simulink model "Final_System_Model_V10"  (R2018a)
settings: Solver=VariableStepAuto  StartTime=0  StopTime=250  FixedStep=0.5  RelTol=1e-3
PreLoadFcn:
  | Ts_Power=1e-6;
  | Ts_Control=100e-6;
undefined symbols (not defined in the file): DiscIntNeverNeededParam, sigbuilder_block
libraries: simulink x24, fl_lib x16, powerlib x15, nesl_utility x8, powerlib_meascontrol x5, re_lib x1
(part 1 of 8)
Description:
  | Copyright 2008-2017 The MathWorks, Inc.
settings Model: SimulationMode=accelerator  PacingRate=0.001000  Creator=MathWorks  LastModifiedBy=Mina
settings SolverCC: ZeroCrossControl=EnableAll  ZeroCrossAlgorithm=Adaptive  AlgebraicLoopSolver=LineSearch
settings DataIOCC: LimitDataPoints=on  SaveFormat=Array  SignalLoggingSaveFormat=ModelDataLogs  SignalLogging=off  DSMLogging=off
settings OptimizationCC: ExpressionDepthLimit=2147483647  LifeSpan=inf
settings DebuggingCC: SolverPrmCheckMsg=warning  FcnCallInpInsideContextMsg=warning  StateNameClashWarn=warning  SFUnexpectedBacktrackingDiag=warning  SFNoUnconditionalDefaultTransitionDiag=warning  SFExecutionAtInitializationDiag=none
settings HardwareCC: ProdBitPerPointer=32  ProdBitPerSizeT=32  ProdBitPerPtrDiffT=32  ProdLargestAtomicFloat=None  ProdIntDivRoundTo=Undefined  ProdEndianess=Unspecified  ProdWordSize=32  ProdHWDeviceType=32-bit Generic
settings ModelReferenceCC: PropagateSignalLabelsOutOfModel=off
settings CodeAppCC: StateflowObjectComments=on
settings GRTTargetCC: TargetLangStandard=C89/C90 (ANSI)  GeneratePreprocessorConditionals=Disable all  CombineOutputUpdateFcns=off  GRTInterface=on
settings ConfigComp: CovMetricSettings=dw  CovHtmlReporting=on  CovSaveCumulativeToWorkspaceVar=on  CovSaveSingleToWorkspaceVar=on  CovExternalEMLEnable=off  CovSFcnEnable=off
settings SimscapeCC: SimscapeNormalizeSystem=off

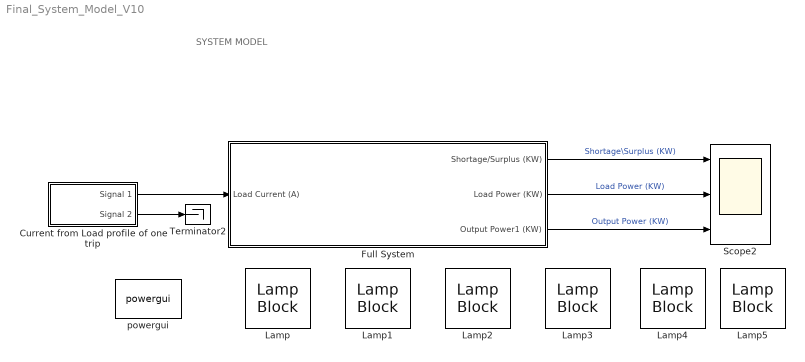
== system Final_System_Model_V10 ==
  note: SYSTEM MODEL
  Current from Load profile of one trip : Subsystem  Tag=STV Subsys  LoadFcn=sigbuilder_block('load');  StartFcn=sigbuilder_block('start');  StopFcn=sigbuilder_block('stop');  ClipboardFcn=sigbuilder_block('clipboard');  mask(Sigbuilder block){tuvar=[0:10]}
      mask help: Simulink:masks:SigbuilderBlock_MD
      mask init:
      | if ~strcmp(get_param(bdroot(gcbh),'SimulationStatus'),'stopped') tuvar = sigbuilder_block('maskInit'); end
      settings: CopyFcn=sigbuilder_block('copy');  DeleteFcn=sigbuilder_block('delete');  ModelCloseFcn=sigbuilder_block('modelClose');  PreSaveFcn=sigbuilder_block('preSave');  PauseFcn=sigbuilder_block('pause');  ContinueFcn=sigbuilder_block('continue');  NameChangeFcn=sigbuilder_block('namechange');  OpenFcn=sigbuilder_block('open',[403.5 117 550.5 359.25 ]);  CloseFcn=sigbuilder_block('close');
      mask Display: plot(0, 0, 100, 100,[2, 2, 32, 32, 2], [68, 8, 8, 68, 68],[32, 2], [38, 38], [32, 19, 2],[53, 60, 44], [32, 17, 17, 2],[16, 16, 31, 31]);txt = getActiveGroup(gcbh);text(2, 100, txt,'verticalAlignment', 'top');
  Full System : Subsystem
  Lamp : LampBlock  WebBlockId=4884
  Lamp1 : LampBlock  WebBlockId=4889
  Lamp2 : LampBlock  WebBlockId=4890
  Lamp3 : LampBlock  WebBlockId=4891
  Lamp4 : LampBlock  WebBlockId=4892
  Lamp5 : LampBlock  WebBlockId=4893
  Scope2 : Scope  NumInputPorts=3
  Terminator2 : Terminator
  powergui : powerlib/powergui  Priority=1  SimulationMode=Discrete  SampleTime=5e-5  frequency=60  Iterations=50  frequencyindice=0  Pbase=100e6  ErrMax=1e-4  UnitsV=kV  UnitsW=MW  buscounter=0  FunctionMessages=off  echomessages=off  EnableUseOfTLC=off  CurrentSourceSwitches=off  DisableSnubberDevices=off  DisableRonSwitches=off  DisableVfSwitches=off  DisplayEquations=off  SolverType=Tustin/Backward Euler (TBE)  Interpol=off  ExternalGateDelay=off  methode=off  Ts=100  x0status=blocks  SPID=off  SwTol=0  HookPort=off  RestoreLinks=warning  ResistiveCurrentMeasurement=off  Frange=[0:2:500]  Ylog=off  Xlog=on  ShowGrid=off  save=off  variable=ZData  structure=0  ZoomFFT=off  StartTime=0.0  cycles=1  DisplayStyle=1  fundamental=60  FreqAxis=off  MaxFrequency=1000  frequencyindicesteady=1  RmsSteady=1  display=off
  wires:
  Current from Load profile of one trip/1(Signal 1) -> Full System/1(Load Current (A))
  Current from Load profile of one trip/2(Signal 2) -> Terminator2/1
  Full System/1(Shortage/Surplus (KW)) -> Scope2/1  "Shortage\\Surplus (KW)"
  Full System/2(Load Power (KW)) -> Scope2/2  "Load Power (KW)"
  Full System/3(Output Power1 (KW)) -> Scope2/3  "Output Power (KW)"

== system Final_System_Model_V10/Current from Load profile of one trip ==
  Demux : Demux  Tag=STV Demux  Outputs=2
  FromWs : FromWorkspace  Tag=STV FromWs  VariableName=tuvar  SampleTime=0
      SigBuilderData=|
      | common.afterFinalStr = 'Extrapolate'
      | common.sampleTime = 0
      | dataSet.timeRange = [0 300]
      | dataSet.name = 'Group 1'
      | sbobj.Groups.Name = 'Group 1'
      | sbobj.Groups.Signals(1).Name = 'Signal 1'
      | sbobj.Groups.Signals(1).XData = [0 2.75 2.75 5.75 5.75 10.98 10.98 24 24 24.6 24.6 27.61 27.61 30.61 30.61 33.73 33.73 36.73 48 48 52.19 52.19 55.19 55.19 59.38 59.38 62.38 72 72 84 84 96 96 108 108 120 120 132 132 144 144 146.76 146.76 147.76 147.76 156 156 168 168 175.76 175.76 176.76 176.76 180 180 192 192 204 204 216 216 216.76 216.76 217.76 217.76 228 228 240 240 244.83 244.83 300]
      | sbobj.Groups.Signals(1).YData = [145.4545455 145.4545455 0.01 0.01 145.4545455 145.4545455 0.01 0.01 195.4545455 195.4545455 486.3636364 486.3636364 0.01 0.01 404.5454545 404.5454545 0.01 0.01 0.01 486.3636364 486.3636364 0.01 0.01 486.3636364 486.3636364 0.01 0.01 0.01 463.6363636 463.6363636 0.01 0.01 463.6363636 463.6363636 0.01 0.01 463.6363636 463.6363636 0.01 0.01 463.6363636 463.6363636 0.01 0.01 463.6363636 463.6363636 0.01 0.01 463.6363636 463.6363636 0.01 0.01 463.6363636 463.6363636 0.01 0.01 463.6363636 463.6363636 0.01 0.01 463.6363636 463.6363636 0.01 0.01 463.6363636 463.6363636 0.01 0.01 463.6363636 463.6363636 0.01 0.01]
      | sbobj.Groups.Signals(2).Name = 'Signal 2'
      | sbobj.Groups.Signals(2).XData = [0 300]
      | sbobj.Groups.Signals(2).YData = [243 243]
      | sbobj.Groups.TimeRange = [0 300]
  Signal 1 : Outport  Tag=STV Outport
  Signal 2 : Outport  Tag=STV Outport  Port=2
  wires:
  Demux/2 -> Signal 2/1
  FromWs/1 -> Demux/1
  Demux/1 -> Signal 1/1

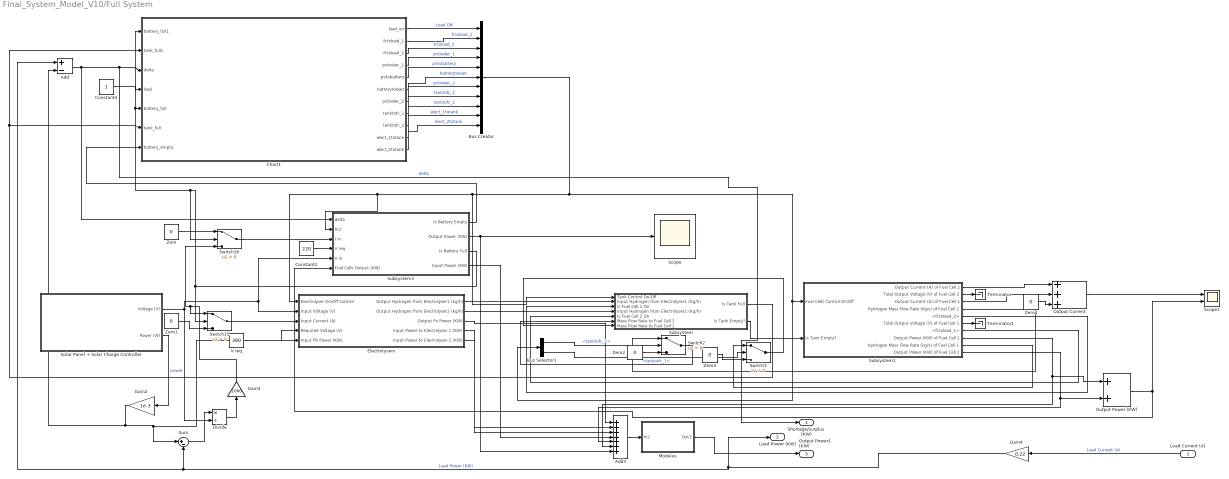
== system Final_System_Model_V10/Full System ==
  Load Current (A) : Inport
  Add : Sum  Inputs=+-
  Add3 : Sum  Inputs=+++++++
  Bus Creator : BusCreator  Inputs=11
  Bus Selector1 : BusSelector  OutputSignals=tanktofc_2,tanktofc_1
  Chart1 : Stateflow chart  TreatAsAtomicUnit=on
  Constant2 : Constant  Value=220
  Constant4 : Constant
  Divide : Product  Inputs=*/
  Electrolysers : Subsystem
  Gain2 : Gain  Gain=1e-3
  Gain3 : Gain  Gain=1000
  Gain4 : Gain  Gain=0.22
  Modulus : Subsystem
  Output Current : Sum  Inputs=+++
  Output Power (KW) : Sum
  Scope : Scope
  Scope1 : Scope  NumInputPorts=2
  Solar Panel + Solar Charge Controller : Subsystem
  Subsystem : Subsystem
  Subsystem1 : Subsystem
  Subsystem3 : Subsystem
  Sum : Sum  Inputs=|+-
  Switch{2..3,15..16} (4 alike) : Switch  Criteria=u2 > Threshold
  Terminator : Terminator
  Terminator1 : Terminator
  V req : Constant  Value=380
  Zero{,1..4} (5 alike) : Constant  Value=0
  Shortage/Surplus (KW) : Outport
  Load Power (KW) : Outport  Port=2
  Output Power1 (KW) : Outport  Port=3
  wires:
  Chart1/5(pvtobattery) -> Bus Creator/5  "pvtobattery"
  Gain2/1 -> Sum/1, Electrolysers/5(Input PV Power (KW)), Add/2
  Subsystem1/1(Output Current (A) of Fuel Cell 2) -> Output Current/1
  Subsystem3/4(Input Power (KW)) -> Add3/4
  Subsystem1/8(Output Power (KW) of Fuel Cell 1) -> Add3/6, Output Power (KW)/1
  Solar Panel + Solar Charge Controller/1(Voltage (V)) -> Subsystem3/5(V in), Electrolysers/2(Input Voltage (V)), Divide/2
  Subsystem/1(Is Tank Full) -> Chart1/2(tank_full1), Chart1/6(tank_full)
  Output Current/1 -> Scope1/1
  Subsystem3/2(Output Power (KW)) -> Scope/1, Add3/7
  Output Power (KW)/1 -> Subsystem3/6(Fuel Cells Output (KW)), Scope1/2
  Bus Creator/1 -> Subsystem3/2(In2), Electrolysers/1(Electrolyser On/Off Control), Subsystem/1(Tank Control On/Off), Bus Selector1/1, Subsystem1/1(Fuel Cells Control On/Off)
  Chart1/9(tanktofc_2) -> Bus Creator/9  "tanktofc_2"
  Zero2/1 -> Switch2/3
  Gain4/1 -> Load Power (KW)/1, Sum/2, Add/1  "Load Power (KW)"
  Gain3/1 -> Switch16/3, Switch15/1
  Subsystem1/6(Total Output Voltage (V) of Fuel Cell 1) -> Terminator1/1
  Chart1/7(pvtoelec_2) -> Bus Creator/7  "pvtoelec_2"
  Zero/1 -> Switch16/1
  V req/1 -> Electrolysers/4(Required Voltage (V))
  Chart1/10(elect_1totank) -> Bus Creator/10  "elect_1totank"
  Add3/1 -> Modulus/1(In1)
  Subsystem1/10(Output Power (KW) of Fuel Cell 2) -> Output Power (KW)/2, Add3/5
  Add/1 -> Shortage/Surplus (KW)/1, Chart1/3(delta), Subsystem3/1(delta)  "delta"
  Electrolysers/2(Output Hydrogen from Electrolyser2 (kg/h)) -> Subsystem/4(Input Hydrogen from Electrolyser2 (Kg/h))
  Divide/1 -> Gain3/1
  Subsystem1/3(Output Current (A) of Fuel Cell 1) -> Output Current/2
  Chart1/6(batterytoload) -> Bus Creator/6  "batterytoload"
  Chart1/3(fctoload_2) -> Bus Creator/3  "fctoload_2"
  Subsystem1/9(Hydrogen Mass Flow Rate (kg/s) of Fuel Cell 1) -> Switch3/1
  Subsystem3/3("Is Battery Full ") -> Switch16/2, Chart1/1(battery_full1), Chart1/5(battery_full), Switch15/2
  Subsystem1/4(Hydrogen Mass Flow Rate (kg/s) of Fuel Cell 2) -> Switch2/1
  Chart1/2(fctoload_1) -> Bus Creator/2  "fctoload_1"
  Load Current (A)/1 -> Gain4/1  "Load Current (A)"
  Subsystem1/5(<fctoload_2>) -> Subsystem/3(Is Fuel Cell 1 On)
  Constant2/1 -> Subsystem3/4(V req)
  Electrolysers/1(Output Hydrogen from Electrolyser1 (kg/h)) -> Subsystem/2(Input Hydrogen from Electrolyser1 (Kg/h))
  Switch3/1 -> Subsystem/7(Mass Flow Rate to Fuel Cell 1)
  Subsystem3/1(Is Battery Empty) -> Chart1/7(battery_empty)
  Solar Panel + Solar Charge Controller/2(Power (W)) -> Gain2/1  "power"
  Zero4/1 -> Output Current/3
  Bus Selector1/1 -> Switch2/2  "<tanktofc_2>"
  Switch2/1 -> Subsystem/6(Mass Flow Rate to Fuel Cell 2)
  Constant4/1 -> Chart1/4(load)
  Chart1/8(tanktofc_1) -> Bus Creator/8  "tanktofc_1"
  Subsystem/2(Is Tank Empty?) -> Subsystem1/2(Is Tank Empty?)
  Zero3/1 -> Switch3/3
  Electrolysers/3(Output Pv Power (KW)) -> Add3/1
  Subsystem1/7(<fctoload_1>) -> Subsystem/5(Is Fuel Cell 2 On)
  Electrolysers/5(Input Power to Electrolyser 2 (KW)) -> Add3/3
  Modulus/1(Out1) -> Output Power1 (KW)/1
  Switch16/1 -> Subsystem3/3(I in)
  Chart1/4(pvtoelec_1) -> Bus Creator/4  "pvtoelec_1"
  Bus Selector1/2 -> Switch3/2  "<tanktofc_1>"
  Chart1/1(load_on) -> Bus Creator/1  "Load ON"
  Chart1/11(elect_2totank) -> Bus Creator/11  "elect_2totank"
  Sum/1 -> Divide/1
  Switch15/1 -> Electrolysers/3(Input Current (A))
  Electrolysers/4(Input Power to Electrolyser 1 (KW)) -> Add3/2
  Subsystem1/2(Total Output Voltage (V) of Fuel Cell 2) -> Terminator/1
  Zero1/1 -> Switch15/3

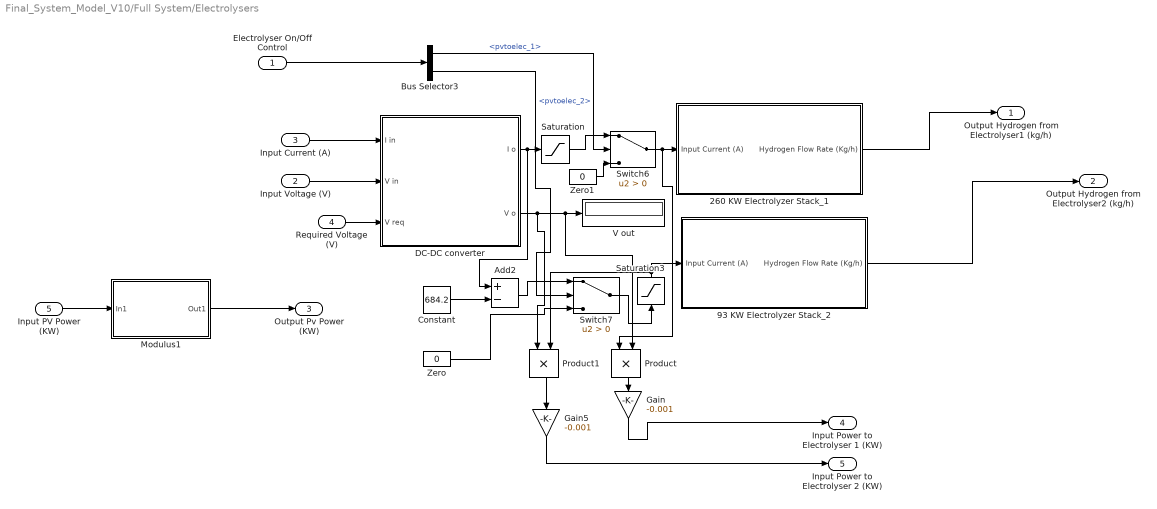
== system Final_System_Model_V10/Full System/Electrolysers ==
  Electrolyser On/Off Control : Inport
  Input Voltage (V) : Inport  Port=2
  Input Current (A) : Inport  Port=3
  Required Voltage (V) : Inport  Port=4
  Input PV Power (KW) : Inport  Port=5
  260 KW Electrolyzer Stack_1 : Subsystem
  93 KW Electrolyzer Stack_2 : Subsystem
  Add2 : Sum  Inputs=+-
  Bus Selector3 : BusSelector  OutputSignals=pvtoelec_1,pvtoelec_2
  Constant : Constant  Value=684.2
  DC-DC converter : Subsystem
  Gain : Gain  Gain=-0.001
  Gain5 : Gain  Gain=-0.001
  Modulus1 : Subsystem
  Product : Product
  Product1 : Product
  Saturation : Saturate  UpperLimit=684.2  LowerLimit=0
  Saturation3 : Saturate  UpperLimit=inf  LowerLimit=0
  Switch6 : Switch  Criteria=u2 > Threshold
  Switch7 : Switch  Criteria=u2 > Threshold
  V out : Display
  Zero : Constant  Value=0
  Zero1 : Constant  Value=0
  Output Hydrogen from Electrolyser1 (kg/h) : Outport
  Output Hydrogen from Electrolyser2 (kg/h) : Outport  Port=2
  Output Pv Power (KW) : Outport  Port=3
  Input Power to Electrolyser 1 (KW) : Outport  Port=4
  Input Power to Electrolyser 2 (KW) : Outport  Port=5
  wires:
  Add2/1 -> Switch7/1
  Switch7/1 -> Saturation3/1
  Bus Selector3/1 -> Switch6/2  "<pvtoelec_1>"
  Required Voltage (V)/1 -> DC-DC converter/3(V req)
  DC-DC converter/2(V o) -> Product1/1, Product/2, V out/1
  Electrolyser On/Off Control/1 -> Bus Selector3/1
  Constant/1 -> Add2/2
  Saturation3/1 -> Product1/2, 93 KW Electrolyzer Stack_2/1(Input Current (A))
  Bus Selector3/2 -> Switch7/2  "<pvtoelec_2>"
  Switch6/1 -> Product/1, 260 KW Electrolyzer Stack_1/1(Input Current (A))
  DC-DC converter/1(I o) -> Add2/1, Saturation/1
  Product1/1 -> Gain5/1
  Gain/1 -> Input Power to Electrolyser 1 (KW)/1
  Product/1 -> Gain/1
  Zero1/1 -> Switch6/3
  Input PV Power (KW)/1 -> Modulus1/1(In1)
  Saturation/1 -> Switch6/1
  260 KW Electrolyzer Stack_1/1(Hydrogen Flow Rate (Kg/h)) -> Output Hydrogen from Electrolyser1 (kg/h)/1
  Input Voltage (V)/1 -> DC-DC converter/2(V in)
  Gain5/1 -> Input Power to Electrolyser 2 (KW)/1
  Input Current (A)/1 -> DC-DC converter/1(I in)
  Modulus1/1(Out1) -> Output Pv Power (KW)/1
  93 KW Electrolyzer Stack_2/1(Hydrogen Flow Rate (Kg/h)) -> Output Hydrogen from Electrolyser2 (kg/h)/1
  Zero/1 -> Switch7/3

== system Final_System_Model_V10/Full System/Modulus ==
  In1 : Inport
  Gain7 : Gain  Gain=-1
  Switch14 : Switch
  Out1 : Outport
  wires:
  In1/1 -> Switch14/1, Switch14/2, Gain7/1
  Gain7/1 -> Switch14/3
  Switch14/1 -> Out1/1

== system Final_System_Model_V10/Full System/Solar Panel + Solar Charge Controller ==
  Mux : Mux  Inputs=2
  Number of modules : Constant  Value=480
  PV Insert inputs here : Subsystem
      mask Display: image('C:\Users\Kimo Store\Desktop\PV Simulink\pva.jpg');
  PV Array : re_lib/Solar/PV Array  Commented=on  Npar=240  Nser=2  PlotType=array @ 1000 W/m2 & specified temperatures  S_vec="[ 1000  250 ]"  Temp_C_vec="[0 25 50  ]"  ModuleName=SunPower SPR-X21-345-COM  PlotWhenSelected=off  Pm=344.946  Ncell=96  Voc=68.2  Isc=6.39  Vm=57.3  Im=6.02  beta_Voc_pc=-0.356  alpha_Isc_pc=0.07  beta_Voc=-0.24279  alpha_Isc=0.004473  IL=6.3928  I0=1.9084e-10  nI=1.1415  Rsh=884.5543  Rs=0.39387  BAL=on  Tc=5e-7  Tfilter=5e-5
  "Power FN " : Fcn  Expr=u(1)*u(2)
  Scope : Scope  Commented=on  NumInputPorts=3
  Solar Charge Controller : Subsystem  Commented=on
  Solar Charge Controller MPPT it is a device which track a point which has the max power : Subsystem
  System Curves : Scope  NumInputPorts=3
  powergui : powerlib/powergui  Priority=1  SimulationMode=Discrete  SampleTime=50e-6  frequency=60  Iterations=50  frequencyindice=0  Pbase=100e6  ErrMax=1e-4  UnitsV=kV  UnitsW=MW  buscounter=0  FunctionMessages=off  echomessages=off  EnableUseOfTLC=off  CurrentSourceSwitches=off  DisableSnubberDevices=off  DisableRonSwitches=off  DisableVfSwitches=off  DisplayEquations=off  SolverType=Tustin/Backward Euler (TBE)  Interpol=off  ExternalGateDelay=off  methode=off  Ts=100  x0status=blocks  SPID=off  SwTol=0  HookPort=off  RestoreLinks=warning  ResistiveCurrentMeasurement=off  Frange=[0:2:500]  Ylog=off  Xlog=on  ShowGrid=off  save=off  variable=ZData  structure=0  ZoomFFT=off  StartTime=0.0  cycles=1  DisplayStyle=1  fundamental=60  FreqAxis=off  MaxFrequency=1000  frequencyindicesteady=1  RmsSteady=1  display=off
  Voltage (V) : Outport
  Power (W) : Outport  Port=2
  wires:
  PV Array/1 -> Solar Charge Controller/1(m)
  Solar Charge Controller/3(Power) -> Scope/3  "Power"
  Solar Charge Controller/2(Current) -> Scope/2  "I"
  Solar Charge Controller/1(Voltage) -> Scope/1  "V"
  PV Insert inputs here/1(I_PV) -> Solar Charge Controller MPPT it is a device which track a point which has the max power/1(I'_PV)  "PV Current (A)"
  [N] -> Solar Charge Controller MPPT it is a device which track a point which has the max power/2(PV num)
  Solar Charge Controller MPPT it is a device which track a point which has the max power/1(I_PV) -> Mux/1, System Curves/1
  [A] -> PV Insert inputs here/1(V_PV)
  "Power FN "/1 -> Power (W)/1, System Curves/3
  Number of modules/1 -> PV Insert inputs here/2(PV num), [N]
  Mux/1 -> "Power FN "/1
  Solar Charge Controller MPPT it is a device which track a point which has the max power/2("V'_PV ") -> Voltage (V)/1, [A], System Curves/2, Mux/2
  connections:
  PV Array/RConn1 -- Solar Charge Controller/LConn1
  PV Array/RConn2 -- Solar Charge Controller/LConn2

== system Final_System_Model_V10/Full System/Subsystem ==
  Tank Control On/Off : Inport
  Input Hydrogen from Electrolyser1 (Kg/h) : Inport  Port=2
  Is Fuel Cell 1 On : Inport  Port=3
  Input Hydrogen from Electrolyser2 (Kg/h) : Inport  Port=4
  Is Fuel Cell 2 On : Inport  Port=5
  Mass Flow Rate to Fuel Cell 2 : Inport  Port=6
  Mass Flow Rate to Fuel Cell 1 : Inport  Port=7
  Add1 : Sum
  Bus Selector2 : BusSelector  OutputSignals=elect_1totank,elect_2totank
  Display2 : Display
  Gain1 : Gain  Gain=1/3600
  Switch4 : Switch  Criteria=u2 > Threshold
  Switch5 : Switch  Criteria=u2 > Threshold
  Tank : Subsystem
  Tank Control : Subsystem
  Zero : Constant  Value=0
  Zero1 : Constant  Value=0
  Is Tank Full : Outport
  Is Tank Empty? : Outport  Port=2
  wires:
  Add1/1 -> Gain1/1
  Zero/1 -> Switch4/3
  Switch4/1 -> Add1/1
  Tank Control/1(Is Fuel Cell ON) -> Tank/2(Is Fuel Cell ON)
  Zero1/1 -> Switch5/3
  Bus Selector2/2 -> Switch5/2  "<elect_2totank>"
  Bus Selector2/1 -> Switch4/2  "<elect_1totank>"
  Switch5/1 -> Add1/2
  Gain1/1 -> Display2/1, Tank/3(Input Hydrogen From Electrolyzer (Kg/s))  "Kg/s"
  Tank Control On/Off/1 -> Bus Selector2/1
  Tank/1(Tank Empty) -> Is Tank Empty?/1  "Is Tank Empty?"
  Tank/2(tank Full) -> Is Tank Full/1
  Input Hydrogen from Electrolyser2 (Kg/h)/1 -> Switch5/1
  Mass Flow Rate to Fuel Cell 2/1 -> Tank/4(Mass Flow Rate To Fuel Cell_2)
  Mass Flow Rate to Fuel Cell 1/1 -> Tank/1(Mass Flow Rate To Fuel Cell_1)
  Is Fuel Cell 2 On/1 -> Tank Control/2(Is fuel cell on2)
  Is Fuel Cell 1 On/1 -> Tank Control/1(Is fuel cell on1)
  Input Hydrogen from Electrolyser1 (Kg/h)/1 -> Switch4/1

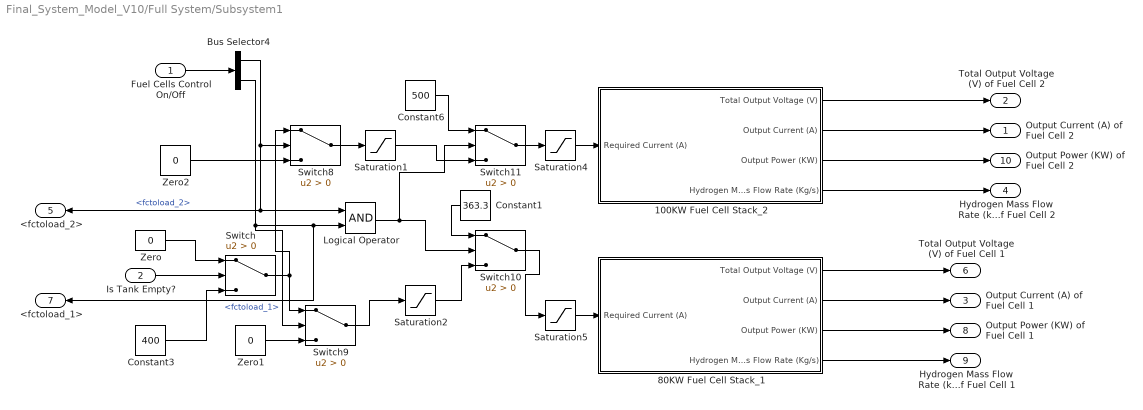
== system Final_System_Model_V10/Full System/Subsystem1 ==
  Fuel Cells Control On/Off : Inport
  Is Tank Empty? : Inport  Port=2
  100KW Fuel Cell Stack_2 : Subsystem
  80KW Fuel Cell Stack_1 : Subsystem
  Bus Selector4 : BusSelector  OutputSignals=fctoload_2,fctoload_1
  Constant1 : Constant  Value=363.3
  Constant3 : Constant  Value=400
  Constant6 : Constant  Value=500
  Logical Operator : Logic  AllPortsSameDT=off  OutDataTypeStr=boolean
  Saturation1 : Saturate  UpperLimit=500  LowerLimit=0
  Saturation2 : Saturate  UpperLimit=400  LowerLimit=0
  Saturation4 : Saturate  UpperLimit=inf  LowerLimit=0
  Saturation5 : Saturate  UpperLimit=inf  LowerLimit=0
  Switch{,8..11} (5 alike) : Switch  Criteria=u2 > Threshold
  Zero : Constant  Value=0
  Zero1 : Constant  Value=0
  Zero2 : Constant  Value=0
  Output Current (A) of Fuel Cell 2 : Outport
  Total Output Voltage (V) of Fuel Cell 2 : Outport  Port=2
  Output Current (A) of Fuel Cell 1 : Outport  Port=3
  Hydrogen Mass Flow Rate (kg/s) of Fuel Cell 2 : Outport  Port=4
  <fctoload_2> : Outport  Port=5
  Total Output Voltage (V) of Fuel Cell 1 : Outport  Port=6
  <fctoload_1> : Outport  Port=7
  Output Power (KW) of Fuel Cell 1 : Outport  Port=8
  Hydrogen Mass Flow Rate (kg/s) of Fuel Cell 1 : Outport  Port=9
  Output Power (KW) of Fuel Cell 2 : Outport  Port=10
  wires:
  Switch10/1 -> Saturation5/1
  Bus Selector4/1 -> Logical Operator/1, <fctoload_2>/1, Switch8/2  "<fctoload_2>"
  Saturation2/1 -> Switch10/3
  Logical Operator/1 -> Switch11/2, Switch10/2
  Zero/1 -> Switch/1
  Saturation5/1 -> 80KW Fuel Cell Stack_1/1(Required Current (A))
  80KW Fuel Cell Stack_1/3(Output Power (KW)) -> Output Power (KW) of Fuel Cell 1/1
  Switch/1 -> Switch9/1, Switch8/1
  Switch9/1 -> Saturation2/1
  Saturation1/1 -> Switch11/3
  Switch8/1 -> Saturation1/1
  Zero2/1 -> Switch8/3
  Constant6/1 -> Switch11/1
  Is Tank Empty?/1 -> Switch/2
  Bus Selector4/2 -> Switch9/2, <fctoload_1>/1, Logical Operator/2  "<fctoload_1>"
  100KW Fuel Cell Stack_2/4(Hydrogen Mass Flow Rate (Kg/s)) -> Hydrogen Mass Flow Rate (kg/s) of Fuel Cell 2/1
  Switch11/1 -> Saturation4/1
  Zero1/1 -> Switch9/3
  Constant1/1 -> Switch10/1
  100KW Fuel Cell Stack_2/3(Output Power (KW)) -> Output Power (KW) of Fuel Cell 2/1
  Constant3/1 -> Switch/3
  80KW Fuel Cell Stack_1/1(Total Output Voltage (V)) -> Total Output Voltage (V) of Fuel Cell 1/1
  Saturation4/1 -> 100KW Fuel Cell Stack_2/1(Required Current (A))
  80KW Fuel Cell Stack_1/4(Hydrogen Mass Flow Rate (Kg/s)) -> Hydrogen Mass Flow Rate (kg/s) of Fuel Cell 1/1
  100KW Fuel Cell Stack_2/2(Output Current (A)) -> Output Current (A) of Fuel Cell 2/1
  80KW Fuel Cell Stack_1/2(Output Current (A)) -> Output Current (A) of Fuel Cell 1/1
  Fuel Cells Control On/Off/1 -> Bus Selector4/1
  100KW Fuel Cell Stack_2/1(Total Output Voltage (V)) -> Total Output Voltage (V) of Fuel Cell 2/1

== system Final_System_Model_V10/Full System/Subsystem3 ==
  delta : Inport
  In2 : Inport  Port=2
  I in : Inport  Port=3
  V req : Inport  Port=4
  V in : Inport  Port=5
  Fuel Cells Output (KW) : Inport  Port=6
  Battery : Subsystem
  Bus Selector : BusSelector  OutputSignals=pvtobattery,batterytoload
  DC-DC converter1 : Subsystem
  Saturation6 : Saturate  UpperLimit=inf  LowerLimit=0
  Subsystem : Subsystem
  Switch1 : Switch  Criteria=u2 > Threshold
  Unit Delay : UnitDelay  SampleTime=-1
  Zero : Constant  Value=0
  Is Battery Empty : Outport
  Output Power (KW) : Outport  Port=2
  "Is Battery Full " : Outport  Port=3
  Input Power (KW) : Outport  Port=4
  wires:
  Switch1/1 -> Saturation6/1
  Bus Selector/2 -> Battery/2(Batterytoload)  "<batterytoload>"
  Saturation6/1 -> Battery/1(Input current1)
  Fuel Cells Output (KW)/1 -> Subsystem/2(Fuel Cells Output (KW))
  V in/1 -> DC-DC converter1/2(V in1)
  Zero/1 -> Switch1/3
  Battery/3(Output Power (KW)) -> Output Power (KW)/1
  Unit Delay/1 -> Switch1/2
  I in/1 -> DC-DC converter1/1(I in1)
  Bus Selector/1 -> Unit Delay/1  "<pvtobattery>"
  Battery/2(Battery Empty1) -> Is Battery Empty/1
  DC-DC converter1/2(I o) -> Switch1/1
  Subsystem/1(Load to battery (KW)) -> Battery/3(Load Power (KW))
  DC-DC converter1/1(V o) -> Battery/4(Input voltage1)
  delta/1 -> Subsystem/1(delta)
  Battery/4(Input Power (KW)) -> Input Power (KW)/1
  V req/1 -> DC-DC converter1/3(V req1)
  In2/1 -> Bus Selector/1
  Battery/1(Battery Full1) -> "Is Battery Full "/1

== system Final_System_Model_V10/Full System/Electrolysers/260 KW Electrolyzer Stack_1 ==
  Input Current (A) : Inport
  Divide : Product  Inputs=*/
  Gain : Gain  Gain=3.6
  H2 flow rate in kg/h : Scope
  Saturation : Saturate  UpperLimit=1.2  LowerLimit=0
  T : Constant  Value=333
  area in cm^2 : Constant  Value=428
  electrolyser stack : Subsystem
  voltage : Scope
  Hydrogen Flow Rate (Kg/h) : Outport
  wires:
  Saturation/1 -> electrolyser stack/2(In2)  "Current Density (A/cm^2)"
  electrolyser stack/2(Out3) -> Gain/1  "H2 flow rate in g/s"
  T/1 -> electrolyser stack/1(In1)
  electrolyser stack/1(Out1) -> voltage/1
  Input Current (A)/1 -> Divide/1
  area in cm^2/1 -> Divide/2
  Divide/1 -> Saturation/1
  Gain/1 -> Hydrogen Flow Rate (Kg/h)/1, H2 flow rate in kg/h/1  "H2 flow rate in kg/h"

== system Final_System_Model_V10/Full System/Electrolysers/93 KW Electrolyzer Stack_2 ==
  Input Current (A) : Inport
  Divide : Product  Inputs=*/
  Gain : Gain  Gain=3.6
  H2 flow rate in kg/h : Scope
  Saturation : Saturate  UpperLimit=1.2  LowerLimit=0
  T : Constant  Value=333
  area in cm^2 : Constant  Value=428
  electrolyser stack : Subsystem
  voltage : Scope
  Hydrogen Flow Rate (Kg/h) : Outport
  wires:
  Gain/1 -> H2 flow rate in kg/h/1, Hydrogen Flow Rate (Kg/h)/1  "H2 flow rate in kg/h"
  Divide/1 -> Saturation/1
  area in cm^2/1 -> Divide/2
  Input Current (A)/1 -> Divide/1
  electrolyser stack/1(Out1) -> voltage/1
  T/1 -> electrolyser stack/1(In1)
  electrolyser stack/2(Out3) -> Gain/1  "H2 flow rate in g/s"
  Saturation/1 -> electrolyser stack/2(In2)  "Current Density (A/cm^2)"

== system Final_System_Model_V10/Full System/Electrolysers/DC-DC converter ==
  I in : Inport
  V in : Inport  Port=2
  V req : Inport  Port=3
  Divide : Product  Inputs=*/
  Product : Product
  Subsystem : Subsystem
  duty cycle : Subsystem
  I o : Outport
  V o : Outport  Port=2
  wires:
  Subsystem/2(V o) -> ?
  V in/1 -> Product/2
  [duty_cycle] -> Subsystem/1(duty cycle)
  Subsystem/1(I o) -> ?
  I in/1 -> Product/1
  Product/1 -> Divide/1
  V req/1 -> V o/1, Divide/2
  Divide/1 -> I o/1

== system Final_System_Model_V10/Full System/Electrolysers/Modulus1 ==
  In1 : Inport
  Gain7 : Gain  Gain=-1
  Switch14 : Switch
  Out1 : Outport
  wires:
  Switch14/1 -> Out1/1
  Gain7/1 -> Switch14/3
  In1/1 -> Gain7/1, Switch14/2, Switch14/1

== system Final_System_Model_V10/Full System/Solar Panel + Solar Charge Controller/PV Insert inputs here ==
  V_PV : Inport
  PV num : Inport  Port=2
  Gain : Gain  Gain=1e-3
  I_sc : Constant  Value=6.39
  Ns_cells : Constant  Value=96
  Product : Product
  Rp : Constant  Value=884.5
  Scope : Scope
  Signal Builder : Subsystem  Tag=STV Subsys  LoadFcn=sigbuilder_block('load');  StartFcn=sigbuilder_block('start');  StopFcn=sigbuilder_block('stop');  ClipboardFcn=sigbuilder_block('clipboard');  mask(Sigbuilder block){tuvar=[0:10]}
      mask help: Simulink:masks:SigbuilderBlock_MD
      mask init:
      | if ~strcmp(get_param(bdroot(gcbh),'SimulationStatus'),'stopped') tuvar = sigbuilder_block('maskInit'); end
      settings: CopyFcn=sigbuilder_block('copy');  DeleteFcn=sigbuilder_block('delete');  ModelCloseFcn=sigbuilder_block('modelClose');  PreSaveFcn=sigbuilder_block('preSave');  PauseFcn=sigbuilder_block('pause');  ContinueFcn=sigbuilder_block('continue');  NameChangeFcn=sigbuilder_block('namechange');  OpenFcn=sigbuilder_block('open',[437.25 153 550.5 359.25 ]);  CloseFcn=sigbuilder_block('close');
      mask Display: plot(0, 0, 100, 100,[2, 2, 32, 32, 2], [68, 8, 8, 68, 68],[32, 2], [38, 38], [32, 19, 2],[53, 60, 44], [32, 17, 17, 2],[16, 16, 31, 31]);txt = getActiveGroup(gcbh);text(2, 100, txt,'verticalAlignment', 'top');
  Subsystem : Subsystem
  Temp : Step  Time=5  Before=25  After=25  SampleTime=0
  V_oc : Constant  Value=68.2
  radiation ratio : Step  Before=1000  After=1000  SampleTime=0
  I_PV : Outport
  wires:
  Subsystem/1(I_PV) -> Scope/1, Product/2  "I_PV(A)"
  Temp/1 -> Subsystem/3(T_o)  "Temperature(c)"
  Signal Builder/1(Signal 1) -> Gain/1  "Radiation ratio"
  Rp/1 -> Subsystem/4(Rp)  "Rp(ohm)"
  V_PV/1 -> Subsystem/1(V_PV)  "V_PV (volt)"
  Product/1 -> I_PV/1
  PV num/1 -> Product/1
  I_sc/1 -> Subsystem/5(I_sc)
  Ns_cells/1 -> Subsystem/6(Ns cells)
  V_oc/1 -> Subsystem/7(V_oc)
  Gain/1 -> Subsystem/2(insolation)

== system Final_System_Model_V10/Full System/Solar Panel + Solar Charge Controller/Solar Charge Controller ==
  note: 5 kHz - 500V
      | Boost Converter
  m : Inport
  Bus Selector : BusSelector  OutputSignals=V_PV,I_PV
  C1 : powerlib/Elements/Series RLC Branch  LConnTagsString=__new0  RConnTagsString=__new0  BranchType=C  Resistance=1.0  Inductance=1.0  SetiL0=off  InitialCurrent=0  Capacitance=12000e-06  Setx0=off  InitialVoltage=0  Measurements=None
  C2 : powerlib/Elements/Series RLC Branch  LConnTagsString=__new0  RConnTagsString=__new0  BranchType=C  Resistance=1.0  Inductance=1.0  SetiL0=off  InitialCurrent=0  Capacitance=12000e-06  Setx0=off  InitialVoltage=0  Measurements=None
  C3 : powerlib/Elements/Series RLC Branch  LConnTagsString=__new0  RConnTagsString=__new0  BranchType=C  Resistance=1.0  Inductance=1.0  SetiL0=off  InitialCurrent=0  Capacitance=100e-6  Setx0=off  InitialVoltage=0  Measurements=Branch voltage
  Deblock Converters : Step  Time=.05  SampleTime=0
  Diode1 : powerlib/Power Electronics/Diode  Ron=1e-4  Lon=0  Vf=0  IC=0  UseSnubber=off  Rs=inf  Cs=inf  Measurements=off
  IGBT1 : powerlib/Power Electronics/IGBT  Ron=0.001  Lon=0  Vf=0  Tf=0  Tt=0  IC=0  Rs=1e5  Cs=inf  Measurements=off
  L1 : powerlib/Elements/Series RLC Branch  LConnTagsString=__new0  RConnTagsString=__new0  BranchType=RL  Resistance=0.005  Inductance=5e-3  SetiL0=off  InitialCurrent=0  Capacitance=1e-6  Setx0=off  InitialVoltage=0  Measurements=None
  "MPPT Controller using  \"Incremental Conductance + Integral Regulator \"  technique " : Subsystem  mask(Boost Control - MPPT){fc=5000, T_MPPT=200e-6, Dinit=0.5}
      mask prompts: fc "PWM switching frequency (Hz)"; T_MPPT "Time window used by MPPT control (s)"; Dinit "Initial value of duty cycle"
  Product : Product
  Product2 : Product  RndMeth=Zero
  "+ " : PMIOPort  Side=Left
  - : PMIOPort  Port=2  Side=Left
  Voltage : Outport
  Current : Outport  Port=2
  Power : Outport  Port=3
  wires:
  Product2/1 -> IGBT1/1
  "MPPT Controller using  \"Incremental Conductance + Integral Regulator \"  technique "/1(Pulses) -> Product2/2
  Deblock Converters/1 -> Product2/1
  Bus Selector/2 -> Product/2, Current/1, "MPPT Controller using  \"Incremental Conductance + Integral Regulator \"  technique "/2(I_PV)  "<I_PV>"
  Bus Selector/1 -> Product/1, Voltage/1, "MPPT Controller using  \"Incremental Conductance + Integral Regulator \"  technique "/1(V_PV)  "<V_PV>"
  m/1 -> Bus Selector/1
  Product/1 -> Power/1
  connections:
  C2/LConn1 -- C1/RConn1
  C3/LConn1 -- "+ "/RConn1 -- L1/LConn1
  C1/LConn1 -- Diode1/RConn1
  L1/RConn1 -- Diode1/LConn1 -- IGBT1/LConn1
  C2/RConn1 -- IGBT1/RConn1 -- C3/RConn1 -- -/RConn1

== system Final_System_Model_V10/Full System/Solar Panel + Solar Charge Controller/Solar Charge Controller MPPT it is a device which track a point which has the max power ==
  I'_PV : Inport
  PV num : Inport  Port=2
  Divide : Product  Inputs=*/
  "MPPT " : Subsystem
  I_PV : Outport
  "V'_PV " : Outport  Port=2
  wires:
  "MPPT "/1(V_mpp) -> "V'_PV "/1, "MPPT "/2(V_PV)  "V_PV(Volt)"
  I'_PV/1 -> I_PV/1, Divide/1
  Divide/1 -> "MPPT "/1(I_PV)
  PV num/1 -> Divide/2

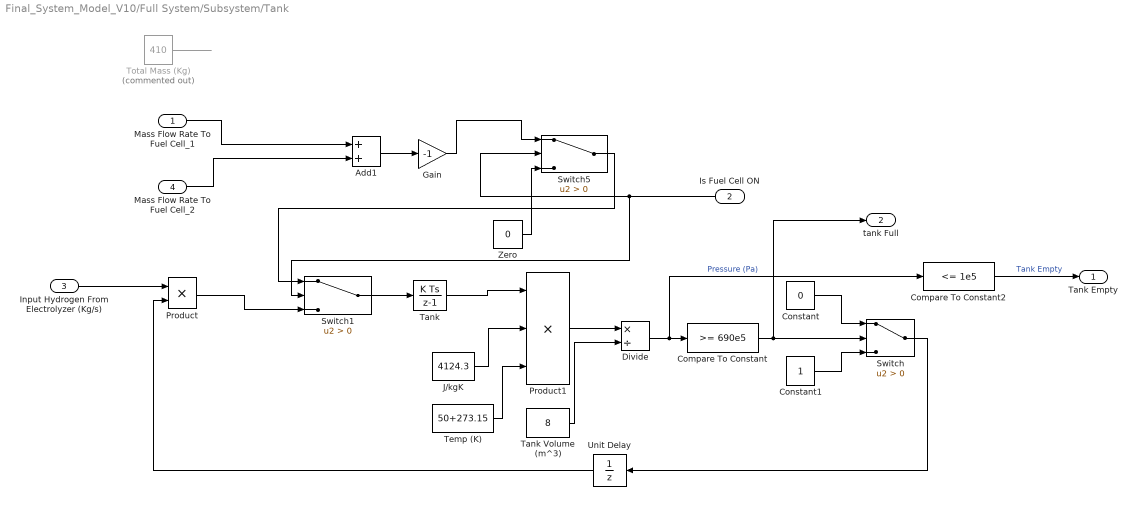
== system Final_System_Model_V10/Full System/Subsystem/Tank ==
  Mass Flow Rate To Fuel Cell_1 : Inport
  Is Fuel Cell ON : Inport  Port=2
  Input Hydrogen From Electrolyzer (Kg/s) : Inport  Port=3
  Mass Flow Rate To Fuel Cell_2 : Inport  Port=4
  Add1 : Sum
  Compare To Constant : simulink/Logic and Bit Operations/Compare To Constant  relop=>=  const=690e5  OutDataTypeStr=boolean
  Compare To Constant2 : simulink/Logic and Bit Operations/Compare To Constant  relop=<=  const=1e5  OutDataTypeStr=boolean
  Constant : Constant  Value=0
  Constant1 : Constant
  Divide : Product  Inputs=*/
  Gain : Gain  Gain=-1
  J/kgK : Constant  Value=4124.3
  Product : Product
  Product1 : Product  Inputs=3
  Switch : Switch  Criteria=u2 > Threshold
  Switch1 : Switch  Criteria=u2 > Threshold
  Switch5 : Switch  Criteria=u2 > Threshold
  Tank : DiscreteIntegrator  InitialCondition=73  SampleTime=-1  LimitOutput=on  UpperSaturationLimit=410  LowerSaturationLimit=0  ICPrevOutput=DiscIntNeverNeededParam  ICPrevScaledInput=DiscIntNeverNeededParam
  Tank Volume (m^3) : Constant  Value=8
  Temp (K) : Constant  Value=50+273.15
  Total Mass (Kg) : Constant  Commented=on  Value=410
  Unit Delay : UnitDelay  SampleTime=-1
  Zero : Constant  Value=0
  Tank Empty : Outport
  tank Full : Outport  Port=2
  wires:
  Switch/1 -> Unit Delay/1
  Product1/1 -> Divide/1
  Divide/1 -> Compare To Constant2/1, Compare To Constant/1  "Pressure (Pa)"
  Tank Volume (m^3)/1 -> Divide/2
  Temp (K)/1 -> Product1/3
  J/kgK/1 -> Product1/2
  Constant1/1 -> Switch/3
  Is Fuel Cell ON/1 -> Switch1/2, Switch5/2
  Compare To Constant2/1 -> Tank Empty/1  "Tank Empty"
  Compare To Constant/1 -> tank Full/1, Switch/2
  Constant/1 -> Switch/1
  Zero/1 -> Switch5/3
  Input Hydrogen From Electrolyzer (Kg/s)/1 -> Product/1
  Add1/1 -> Gain/1
  Unit Delay/1 -> Product/2
  Total Mass (Kg)/1 -> ?
  Product/1 -> Switch1/3
  Mass Flow Rate To Fuel Cell_1/1 -> Add1/1
  Mass Flow Rate To Fuel Cell_2/1 -> Add1/2
  Tank/1 -> Product1/1
  Gain/1 -> Switch5/1
  Switch5/1 -> Switch1/1
  Switch1/1 -> Tank/1

== system Final_System_Model_V10/Full System/Subsystem/Tank Control ==
  note: This Block will be connected to the stateflow chart as to control the state of the tank, either it is:
      | a) Charging Only
      | b) Discharging Only
      | Or
      | c) Charging and Discharging at the same time
  Is fuel cell on1 : Inport
  Is fuel cell on2 : Inport  Port=2
  Logical Operator : Logic  Operator=OR  AllPortsSameDT=off  OutDataTypeStr=boolean
  Is Fuel Cell ON : Outport
  wires:
  Logical Operator/1 -> Is Fuel Cell ON/1
  Is fuel cell on1/1 -> Logical Operator/1
  Is fuel cell on2/1 -> Logical Operator/2

== system Final_System_Model_V10/Full System/Subsystem1/100KW Fuel Cell Stack_2 ==
  note: FUEL CELL DYNAMIC MODEL INCLUDING THE FUEL CELL,HYDROGEN/OXYGEN FEED SYTEMS AND BUCK CONVERTER
  Required Current (A) : Inport
  Bus Creator : BusCreator  Inputs=4
  Bus Selector : BusSelector  OutputSignals=|
      | signal3.Cell Output Voltage (V),signal3.Current Density (A/cm^2),Hydrogen Mass Flow Rate (kg/s),signal3.Output Current,Total Output Voltage (V),Required Current
      | (A),signal3.Air Mass Flow Rate (kg/s)
  Constant : Constant  Value=0.001
  Display : Display
  Display1 : Display
  From Load Current and Fuel Cell Output Current (A) to Valve Restriction Area (m^2) : Subsystem
  Fuel Cell Model : Subsystem  mask(Fuel Cell Model){Temperature_c=80, Hydrogen_Pressure_atm=8, Air_Pressure_atm=8, Number_of_cells=208, Cell_Area_cm_squared=4397.14, Alpha_charge_Transfer_Coefficient=0.5, Exchange_Current_Density_i0=0.00000012246, Internal_Resistance_r=0.019, Amplification_Constant_Alpha1=0.085, Limiting_Current_Density_i_l=2, Mass_Transport_Limit_k=1.1, Dynamic_Response=[5 1]}
      mask prompts: Temperature_c "Temperature (c)"; Hydrogen_Pressure_atm "Hydrogen Pressure (atm)"; Air_Pressure_atm "Air Pressure (atm)"; Number_of_cells "Number Of Cells"; Cell_Area_cm_squared "Cell Area (cm^2)"; Alpha_charge_Transfer_Coefficient "Alpha (Charge Transfer Coefficient)"; Exchange_Current_Density_i0 "Exchange Current Density (i_0)(A/cm^2)"; Internal_Resistance_r "Internal Resistance (r)(Ohm)"; Amplification_Constant_Alpha1 "Amplification Constant (Alpha1)"; Limiting_Current_Density_i_l "Limiting Current Density (i_L)(A/cm^2)"; Mass_Transport_Limit_k "Mass Transport Limit (k)"; Dynamic_Response "Cell Dynamic Response (s)"
      mask help:
      | This is a mathematical Fuel Cell dynamic model. It operates under the Following Assumptions:
      | 1-The model is dynamic ,ie, it models the fuel cell behavior with respect to time.
      | 2-Fuel Cell Temperature is Constant.
      | 3-No Excess Hydrogen ,ie, Every Hydrogen molecule that enters the fuel cell Stack reacts to produce electricity.
      | 4-No excess Air.
      | 5-Concentration Losses are not calculated in the Model as we will never approach this region during operation.
      mask TypeOptions Temperature_c:
      | Stack Temperature
      | (C)/Value
      mask TypeOptions Hydrogen_Pressure_atm: Hydrogen Pressure (atm)/Value
      mask TypeOptions Air_Pressure_atm: Air Pressue (atm)/Value
      mask TypeOptions Number_of_cells: Number of Cells/Value
      mask TypeOptions Cell_Area_cm_squared:
      | Cell Area
      | (cm^2)/Value
      mask TypeOptions Alpha_charge_Transfer_Coefficient:
      | From Current Density (A//cm^2)
      | To
      | Overvoltages (V)/Activation Overvoltage/Alpha
      | Charge Transfer Coefficient1/Value
      mask TypeOptions Exchange_Current_Density_i0:
      | From Current Density (A//cm^2)
      | To
      | Overvoltages (V)/Activation Overvoltage/Reference Exchange Current Density
      | (I_0)1/Value
      mask TypeOptions Internal_Resistance_r:
      | From Current Density (A//cm^2)
      | To
      | Overvoltages (V)/Ohmic Overvoltage/Internal Resistance
      | (r)/Value
      mask TypeOptions Amplification_Constant_Alpha1:
      | From Current Density (A//cm^2)
      | To
      | Overvoltages (V)/Concentration Overvoltage/Amplification Constant
      | Alpha2/Value
      mask TypeOptions Limiting_Current_Density_i_l:
      | From Current Density (A//cm^2)
      | To
      | Overvoltages (V)/Concentration Overvoltage/Limiting Current
      | (i_L)1/Value
      mask TypeOptions Mass_Transport_Limit_k:
      | From Current Density (A//cm^2)
      | To
      | Overvoltages (V)/Concentration Overvoltage/Mass Transport Constant
      | (K)1/Value
      mask TypeOptions Dynamic_Response: Cell dynamic/Denominator
      mask DialogControl Operating_Conditions Prompt: Operating Conditions
      mask DialogControl Fuel_Cell_Parameters Prompt: Fuel Cell Parameters
      mask Display: image(imread('power_fuelcell.png'));port_label('output',1,'m');
  Hydrogen Mass Flow Rate (Kg/s) (Hydrogen Feeding System) : Subsystem
  Load : Subsystem
  OutPut Current2 : Display
  OutPut Voltage2 : Display
  "Output " : Scope  NumInputPorts=8
  PID Controller : simulink/Continuous/PID Controller  Controller=PI  TimeDomain=Continuous-time  SampleTime=-1  IntegratorMethod=Forward Euler  FilterMethod=Forward Euler  Form=Parallel  UseFilter=on  ControllerParametersSource=internal  P=0.1  I=0.7  D=0.01  N=100  InitialConditionSource=internal  InitialConditionForIntegrator=0  InitialConditionForFilter=0  ExternalReset=none  LimitOutput=on  UpperSaturationLimit=2.7e-5  LowerSaturationLimit=-inf  LinearizeAsGain=on  AntiWindupMode=none  Kb=1  TrackingMode=off  Kt=1  PParamMin=[]  PParamMax=[]  IParamMin=[]  IParamMax=[]  DParamMin=[]  DParamMax=[]  NParamMin=[]  NParamMax=[]  KbParamMin=[]  KbParamMax=[]  KtParamMin=[]  KtParamMax=[]  POutMin=[]  POutMax=[]  IOutMin=[]  IOutMax=[]  DOutMin=[]  DOutMax=[]  NOutMin=[]  NOutMax=[]  KbOutMin=[]  KbOutMax=[]  KtOutMin=[]  KtOutMax=[]  IntegratorOutMin=[]  IntegratorOutMax=[]  FilterOutMin=[]  FilterOutMax=[]  SumOutMin=[]  SumOutMax=[]  SumI1OutMin=[]  SumI1OutMax=[]  SumI2OutMin=[]  SumI2OutMax=[]  SumI3OutMin=[]  SumI3OutMax=[]  SumDOutMin=[]  SumDOutMax=[]  SaturationOutMin=[]  SaturationOutMax=[]  IntegratorContinuousStateAttributes=''  IntegratorStateMustResolveToSignalObject=off  IntegratorRTWStateStorageClass=Auto  FilterContinuousStateAttributes=''  FilterStateMustResolveToSignalObject=off  FilterRTWStateStorageClass=Auto  DifferentiatorICPrevScaledInput=0  DifferentiatorOutMin=[]  DifferentiatorOutMax=[]  FilterDiffOutCoefMin=[]  FilterDiffOutCoefMax=[]  SumDenOutMin=[]  SumDenOutMax=[]  SumNumOutMin=[]  SumNumOutMax=[]  ReciprocalOutMin=[]  ReciprocalOutMax=[]  DivideOutMin=[]  DivideOutMax=[]  TunerSelectOption=Transfer Function Based (PID Tuner App)
  PS-Simulink Converter : nesl_utility/PS-Simulink Converter  PhysicalDomain=network_engine_domain  SubClassName=ps_output  LeftPortType=input  RightPortType=output  PseudoPeriodic=off  Frequencies=[]  Unit=1  AffineConversion=off
  Product : Product  Inputs=3
  "Restriction Area (m^2) " : Constant  Value=3.5e-6  VectorParams1D=off
  Saturation : Saturate  UpperLimit=2.7e-5  LowerLimit=0
  Sum : Sum  Inputs=|+-
  Valve : ToWorkspace  VariableName=Valve_Opening_Area  SaveFormat=Timeseries  SampleTime=-1
  Total Output Voltage (V) : Outport
  Output Current (A) : Outport  Port=2
  Output Power (KW) : Outport  Port=3
  Hydrogen Mass Flow Rate (Kg/s) : Outport  Port=4
  wires:
  Bus Selector/7 -> "Output "/7  "<Air Mass Flow Rate (kg/s)>"
  Required Current (A)/1 -> Bus Creator/1  "Required Current (A)"
  Product/1 -> Output Power (KW)/1, "Output "/8  "Output Power (KW)"
  From Load Current and Fuel Cell Output Current (A) to Valve Restriction Area (m^2)/2(Valve Opening from Output Current) -> Sum/2  "Valve Opening as dictated by Fuel Cell Output Current (m^2)"
  Bus Selector/4 -> Output Current (A)/1, OutPut Current2/1, Product/1, "Output "/4, From Load Current and Fuel Cell Output Current (A) to Valve Restriction Area (m^2)/2(Output Current)  "<Output Current>"
  PS-Simulink Converter/1 -> Fuel Cell Model/1(Hydrogen Mass Flow Rate (kg/s)), Bus Creator/4  "Hydrogen Mass Flow Rate (kg/s)"
  Bus Selector/1 -> "Output "/1  "<Cell Output Voltage (V)>"
  Constant/1 -> Product/3
  Bus Creator/1 -> From Load Current and Fuel Cell Output Current (A) to Valve Restriction Area (m^2)/1(Load Profile Current (A)), Bus Selector/1  "Load Profile Current (A)"
  Bus Selector/2 -> "Output "/2  "<Current Density (A/cm^2)>"
  Bus Selector/5 -> Total Output Voltage (V)/1, OutPut Voltage2/1, Product/2, "Output "/5  "<Total Output Voltage (V)>"
  Fuel Cell Model/1(Signal) -> Bus Creator/3, Load/1(Signal)
  Load/1(Total Output Voltage (V)) -> Bus Creator/2
  Bus Selector/3 -> "Output "/3  "<Hydrogen Mass Flow Rate (kg/s)>"
  Sum/1 -> PID Controller/1  "Error signal"
  From Load Current and Fuel Cell Output Current (A) to Valve Restriction Area (m^2)/1(Valve Opening) -> Sum/1  "Valve Opening as dictated by Load Current (A)"
  Saturation/1 -> Display/1, Hydrogen Mass Flow Rate (Kg/s) (Hydrogen Feeding System)/1(Restriction Area (m^2))
  "Restriction Area (m^2) "/1 -> Valve/1
  Bus Selector/6 -> "Output "/6  "<Required Current (A)>"
  PID Controller/1 -> Saturation/1, Display1/1
  From Load Current and Fuel Cell Output Current (A) to Valve Restriction Area (m^2)/3(Hydrogen Mass Flow Rate (Kg/s)) -> Hydrogen Mass Flow Rate (Kg/s)/1
  connections:
  PS-Simulink Converter/LConn1 -- Hydrogen Mass Flow Rate (Kg/s) (Hydrogen Feeding System)/RConn1

== system Final_System_Model_V10/Full System/Subsystem1/80KW Fuel Cell Stack_1 ==
  note: FUEL CELL DYNAMIC MODEL INCLUDING THE FUEL CELL,HYDROGEN/OXYGEN FEED SYTEMS AND BUCK CONVERTER
  Required Current (A) : Inport
  Bus Creator : BusCreator  Inputs=4
  Bus Selector : BusSelector  OutputSignals=|
      | signal3.Cell Output Voltage (V),signal3.Current Density (A/cm^2),Hydrogen Mass Flow Rate (kg/s),signal3.Output Current,Total Output Voltage (V),Required Current
      | (A),signal3.Air Mass Flow Rate (kg/s)
  Constant : Constant  Value=0.001
  Display : Display
  Display1 : Display
  From Load Current and Fuel Cell Output Current (A) to Valve Restriction Area (m^2) : Subsystem
  Fuel Cell Model : Subsystem  mask(Fuel Cell Model){Temperature_c=80, Hydrogen_Pressure_atm=8, Air_Pressure_atm=8, Number_of_cells=208, Cell_Area_cm_squared=4397.14, Alpha_charge_Transfer_Coefficient=0.5, Exchange_Current_Density_i0=0.00000012246, Internal_Resistance_r=0.019, Amplification_Constant_Alpha1=0.085, Limiting_Current_Density_i_l=2, Mass_Transport_Limit_k=1.1, Dynamic_Response=[5 1]}
      mask prompts: Temperature_c "Temperature (c)"; Hydrogen_Pressure_atm "Hydrogen Pressure (atm)"; Air_Pressure_atm "Air Pressure (atm)"; Number_of_cells "Number Of Cells"; Cell_Area_cm_squared "Cell Area (cm^2)"; Alpha_charge_Transfer_Coefficient "Alpha (Charge Transfer Coefficient)"; Exchange_Current_Density_i0 "Exchange Current Density (i_0)(A/cm^2)"; Internal_Resistance_r "Internal Resistance (r)(Ohm)"; Amplification_Constant_Alpha1 "Amplification Constant (Alpha1)"; Limiting_Current_Density_i_l "Limiting Current Density (i_L)(A/cm^2)"; Mass_Transport_Limit_k "Mass Transport Limit (k)"; Dynamic_Response "Cell Dynamic Response (s)"
      mask help:
      | This is a mathematical Fuel Cell dynamic model. It operates under the Following Assumptions:
      | 1-The model is dynamic ,ie, it models the fuel cell behavior with respect to time.
      | 2-Fuel Cell Temperature is Constant.
      | 3-No Excess Hydrogen ,ie, Every Hydrogen molecule that enters the fuel cell Stack reacts to produce electricity.
      | 4-No excess Air.
      | 5-Concentration Losses are not calculated in the Model as we will never approach this region during operation.
      mask TypeOptions Temperature_c:
      | Stack Temperature
      | (C)/Value
      mask TypeOptions Hydrogen_Pressure_atm: Hydrogen Pressure (atm)/Value
      mask TypeOptions Air_Pressure_atm: Air Pressue (atm)/Value
      mask TypeOptions Number_of_cells: Number of Cells/Value
      mask TypeOptions Cell_Area_cm_squared:
      | Cell Area
      | (cm^2)/Value
      mask TypeOptions Alpha_charge_Transfer_Coefficient:
      | From Current Density (A//cm^2)
      | To
      | Overvoltages (V)/Activation Overvoltage/Alpha
      | Charge Transfer Coefficient1/Value
      mask TypeOptions Exchange_Current_Density_i0:
      | From Current Density (A//cm^2)
      | To
      | Overvoltages (V)/Activation Overvoltage/Reference Exchange Current Density
      | (I_0)1/Value
      mask TypeOptions Internal_Resistance_r:
      | From Current Density (A//cm^2)
      | To
      | Overvoltages (V)/Ohmic Overvoltage/Internal Resistance
      | (r)/Value
      mask TypeOptions Amplification_Constant_Alpha1:
      | From Current Density (A//cm^2)
      | To
      | Overvoltages (V)/Concentration Overvoltage/Amplification Constant
      | Alpha2/Value
      mask TypeOptions Limiting_Current_Density_i_l:
      | From Current Density (A//cm^2)
      | To
      | Overvoltages (V)/Concentration Overvoltage/Limiting Current
      | (i_L)1/Value
      mask TypeOptions Mass_Transport_Limit_k:
      | From Current Density (A//cm^2)
      | To
      | Overvoltages (V)/Concentration Overvoltage/Mass Transport Constant
      | (K)1/Value
      mask TypeOptions Dynamic_Response: Cell dynamic/Denominator
      mask DialogControl Operating_Conditions Prompt: Operating Conditions
      mask DialogControl Fuel_Cell_Parameters Prompt: Fuel Cell Parameters
      mask Display: image(imread('power_fuelcell.png'));port_label('output',1,'m');
  Hydrogen Mass Flow Rate (Kg/s) (Hydrogen Feeding System) : Subsystem
  Load : Subsystem
  OutPut Current2 : Display
  OutPut Voltage2 : Display
  "Output " : Scope  NumInputPorts=8
  PID Controller : simulink/Continuous/PID Controller  Controller=PI  TimeDomain=Continuous-time  SampleTime=-1  IntegratorMethod=Forward Euler  FilterMethod=Forward Euler  Form=Parallel  UseFilter=on  ControllerParametersSource=internal  P=0.1  I=0.7  D=0.01  N=100  InitialConditionSource=internal  InitialConditionForIntegrator=0  InitialConditionForFilter=0  ExternalReset=none  LimitOutput=on  UpperSaturationLimit=2.7e-5  LowerSaturationLimit=-inf  LinearizeAsGain=on  AntiWindupMode=none  Kb=1  TrackingMode=off  Kt=1  PParamMin=[]  PParamMax=[]  IParamMin=[]  IParamMax=[]  DParamMin=[]  DParamMax=[]  NParamMin=[]  NParamMax=[]  KbParamMin=[]  KbParamMax=[]  KtParamMin=[]  KtParamMax=[]  POutMin=[]  POutMax=[]  IOutMin=[]  IOutMax=[]  DOutMin=[]  DOutMax=[]  NOutMin=[]  NOutMax=[]  KbOutMin=[]  KbOutMax=[]  KtOutMin=[]  KtOutMax=[]  IntegratorOutMin=[]  IntegratorOutMax=[]  FilterOutMin=[]  FilterOutMax=[]  SumOutMin=[]  SumOutMax=[]  SumI1OutMin=[]  SumI1OutMax=[]  SumI2OutMin=[]  SumI2OutMax=[]  SumI3OutMin=[]  SumI3OutMax=[]  SumDOutMin=[]  SumDOutMax=[]  SaturationOutMin=[]  SaturationOutMax=[]  IntegratorContinuousStateAttributes=''  IntegratorStateMustResolveToSignalObject=off  IntegratorRTWStateStorageClass=Auto  FilterContinuousStateAttributes=''  FilterStateMustResolveToSignalObject=off  FilterRTWStateStorageClass=Auto  DifferentiatorICPrevScaledInput=0  DifferentiatorOutMin=[]  DifferentiatorOutMax=[]  FilterDiffOutCoefMin=[]  FilterDiffOutCoefMax=[]  SumDenOutMin=[]  SumDenOutMax=[]  SumNumOutMin=[]  SumNumOutMax=[]  ReciprocalOutMin=[]  ReciprocalOutMax=[]  DivideOutMin=[]  DivideOutMax=[]  TunerSelectOption=Transfer Function Based (PID Tuner App)
  PS-Simulink Converter : nesl_utility/PS-Simulink Converter  PhysicalDomain=network_engine_domain  SubClassName=ps_output  LeftPortType=input  RightPortType=output  PseudoPeriodic=off  Frequencies=[]  Unit=1  AffineConversion=off
  Product : Product  Inputs=3
  "Restriction Area (m^2) " : Constant  Value=3.5e-6  VectorParams1D=off
  Saturation : Saturate  UpperLimit=2.7e-5  LowerLimit=0
  Sum : Sum  Inputs=|+-
  Valve : ToWorkspace  VariableName=Valve_Opening_Area_1  SaveFormat=Timeseries  SampleTime=-1
  Total Output Voltage (V) : Outport
  Output Current (A) : Outport  Port=2
  Output Power (KW) : Outport  Port=3
  Hydrogen Mass Flow Rate (Kg/s) : Outport  Port=4
  wires:
  From Load Current and Fuel Cell Output Current (A) to Valve Restriction Area (m^2)/3(Hydrogen Mass Flow Rate (Kg/s)) -> Hydrogen Mass Flow Rate (Kg/s)/1
  PID Controller/1 -> Display1/1, Saturation/1
  Bus Selector/6 -> "Output "/6  "<Required Current (A)>"
  "Restriction Area (m^2) "/1 -> Valve/1
  Saturation/1 -> Hydrogen Mass Flow Rate (Kg/s) (Hydrogen Feeding System)/1(Restriction Area (m^2)), Display/1
  From Load Current and Fuel Cell Output Current (A) to Valve Restriction Area (m^2)/1(Valve Opening) -> Sum/1  "Valve Opening as dictated by Load Current (A)"
  Sum/1 -> PID Controller/1  "Error signal"
  Bus Selector/3 -> "Output "/3  "<Hydrogen Mass Flow Rate (kg/s)>"
  Load/1(Total Output Voltage (V)) -> Bus Creator/2
  Fuel Cell Model/1(Signal) -> Load/1(Signal), Bus Creator/3
  Bus Selector/5 -> "Output "/5, Product/2, OutPut Voltage2/1, Total Output Voltage (V)/1  "<Total Output Voltage (V)>"
  Bus Selector/2 -> "Output "/2  "<Current Density (A/cm^2)>"
  Bus Creator/1 -> Bus Selector/1, From Load Current and Fuel Cell Output Current (A) to Valve Restriction Area (m^2)/1(Load Profile Current (A))  "Load Profile Current (A)"
  Constant/1 -> Product/3
  Bus Selector/1 -> "Output "/1  "<Cell Output Voltage (V)>"
  PS-Simulink Converter/1 -> Bus Creator/4, Fuel Cell Model/1(Hydrogen Mass Flow Rate (kg/s))  "Hydrogen Mass Flow Rate (kg/s)"
  Bus Selector/4 -> From Load Current and Fuel Cell Output Current (A) to Valve Restriction Area (m^2)/2(Output Current), "Output "/4, Product/1, OutPut Current2/1, Output Current (A)/1  "<Output Current>"
  From Load Current and Fuel Cell Output Current (A) to Valve Restriction Area (m^2)/2(Valve Opening from Output Current) -> Sum/2  "Valve Opening as dictated by Fuel Cell Output Current (m^2)"
  Product/1 -> "Output "/8, Output Power (KW)/1  "Output Power (KW)"
  Required Current (A)/1 -> Bus Creator/1  "Required Current (A)"
  Bus Selector/7 -> "Output "/7  "<Air Mass Flow Rate (kg/s)>"
  connections:
  PS-Simulink Converter/LConn1 -- Hydrogen Mass Flow Rate (Kg/s) (Hydrogen Feeding System)/RConn1
